simulink model "modular_NL_Modell2"  (R2016b)
settings: Solver=VariableStepAuto  StartTime=0.0  StopTime=15  RelTol=1e-3
values from neighbouring files (symbols this model uses):
  L_0 = 0.2    [StartSim.m]
  phi_0 = 0    [StartSim.m]
  r1 = 0.05    [StartSim.m]
  r2 = 0.05    [StartSim.m]
  T1 = 0.05    [StartSim.m]
  T2 = 0.05    [StartSim.m]
  ue1 = 6    [StartSim.m]
  ue2 = 3    [StartSim.m]
  x_0 = 0    [StartSim.m]
libraries: simulink_extras x2
settings Model: Creator=Patrick  LastModifiedBy=Fritz

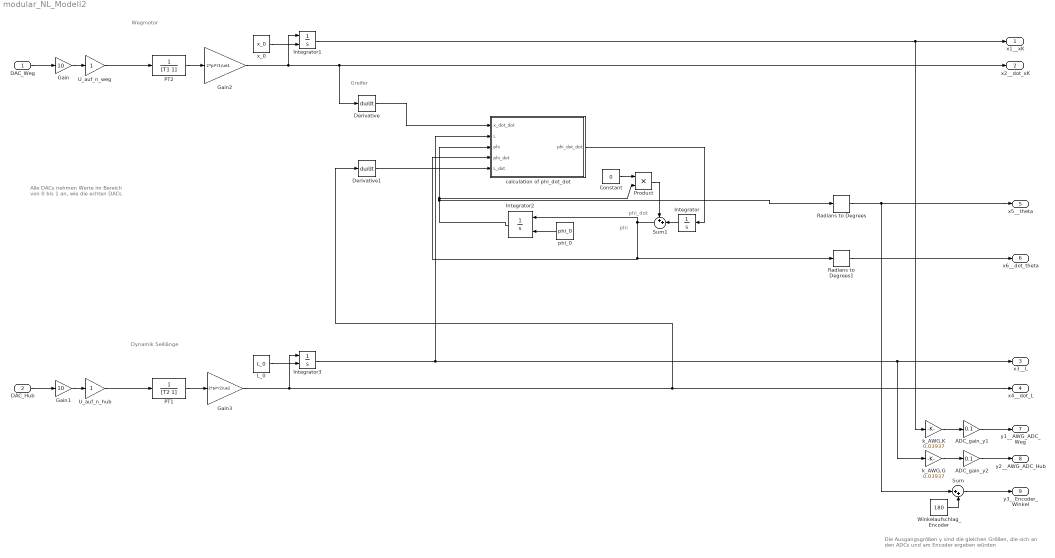
== system modular_NL_Modell2 ==
  note: Greifer
  note: Wegmotor
  note: Dynamik Seillänge
  note: Die Ausgangsgrößen y sind die gleichen Größen,
      | die sich an den ADCs und am Encoder ergeben würden
  note: Alle DACs nehmen Werte im Bereich
      | von 0 bis 1 an, wie die echten DACs
  note: phi_dot
  note: phi
  DAC_Weg : Inport
  DAC_Hub : Inport  Port=2
  ADC_gain_y1 : Gain  Gain=0.1
  ADC_gain_y2 : Gain  Gain=0.1
  Constant : Constant  Value=0
  Derivative : Derivative
  Derivative1 : Derivative
  Gain : Gain  Gain=10
  Gain1 : Gain  Gain=10
  Gain2 : Gain  Gain=2*pi*r1/ue1
  Gain3 : Gain  Gain=2*pi*r2/ue2
  Integrator : Integrator
  Integrator1 : Integrator  InitialConditionSource=external
  Integrator2 : Integrator  InitialConditionSource=external
  Integrator3 : Integrator  InitialConditionSource=external
  L_0 : Constant  Value=L_0
  PT1 : TransferFcn  Denominator=[T2 1]
  PT2 : TransferFcn  Denominator=[T1 1]
  Product : Product
  Radians to Degrees : simulink_extras/Transformations/Radians to Degrees
  Radians to Degrees1 : simulink_extras/Transformations/Radians to Degrees
  Sum : Sum  Inputs=|++
  Sum1 : Sum  Inputs=++|
  U_auf_n_hub : Gain
  U_auf_n_weg : Gain
  Winkelaufschlag_Encoder : Constant  Value=180
  calculation of phi_dot_dot : MATLAB Function  TreatAsAtomicUnit=on
  k_AWG,G : Gain  Gain=0.03937
  k_AWG,K : Gain  Gain=0.03937
  phi_0 : Constant  Value=phi_0
  x_0 : Constant  Value=x_0
  x1__xK : Outport  SignalName=x1__xK
  x2__dot_xK : Outport  Port=2  SignalName=x2__dot_xK
  x3__L : Outport  Port=3  SignalName=x3__L
  x4__dot_L : Outport  Port=4  SignalName=x4__dot_L
  x5__theta : Outport  Port=5  SignalName=x5__theta
  x6__dot_theta : Outport  Port=6  SignalName=x6__dot_theta
  y1__AWG_ADC_Weg : Outport  Port=7  SignalName=y1__AWG_ADC_Weg
  y2__AWG_ADC_Hub : Outport  Port=8  SignalName=y2__AWG_ADC_Hub
  y3__Encoder_Winkel : Outport  Port=9  SignalName=y3__Encoder_Winkel
  wires:
  Integrator2/1 -> calculation of phi_dot_dot/3(phi), Product/2, Radians to Degrees/1
  Sum1/1 -> calculation of phi_dot_dot/4(phi_dot), Radians to Degrees1/1, Integrator2/1
  Radians to Degrees1/1 -> x6__dot_theta/1
  Integrator1/1 -> k_AWG,K/1, x1__xK/1
  Radians to Degrees/1 -> x5__theta/1, Sum/1
  k_AWG,K/1 -> ADC_gain_y1/1
  k_AWG,G/1 -> ADC_gain_y2/1
  Winkelaufschlag_Encoder/1 -> Sum/2
  Sum/1 -> y3__Encoder_Winkel/1
  ADC_gain_y2/1 -> y2__AWG_ADC_Hub/1
  ADC_gain_y1/1 -> y1__AWG_ADC_Weg/1
  DAC_Weg/1 -> Gain/1
  Gain/1 -> U_auf_n_weg/1
  DAC_Hub/1 -> Gain1/1
  Gain1/1 -> U_auf_n_hub/1
  L_0/1 -> Integrator3/2
  PT1/1 -> Gain3/1
  U_auf_n_hub/1 -> PT1/1
  PT2/1 -> Gain2/1
  U_auf_n_weg/1 -> PT2/1
  x_0/1 -> Integrator1/2
  Product/1 -> Sum1/1
  Integrator/1 -> Sum1/2
  Gain2/1 -> x2__dot_xK/1, Derivative/1, Integrator1/1
  Constant/1 -> Product/1
  Gain3/1 -> Integrator3/1, x4__dot_L/1, Derivative1/1
  phi_0/1 -> Integrator2/2
  Derivative1/1 -> calculation of phi_dot_dot/5(L_dot)
  calculation of phi_dot_dot/1(phi_dot_dot) -> Integrator/1
  Integrator3/1 -> k_AWG,G/1, x3__L/1, calculation of phi_dot_dot/2(L)
  Derivative/1 -> calculation of phi_dot_dot/1(x_dot_dot)

== matlab function modular_NL_Modell2/calculation of phi_dot_dot ==
  data: x_dot_dot input; phi_dot_dot output; L input; phi input; phi_dot input; L_dot input
function phi_dot_dot = fcn(x_dot_dot,L,phi,phi_dot,L_dot)

phi_dot_dot = -(cos(phi)/L)*x_dot_dot-9.81/L*sin(phi)-2*L_dot*phi_dot;
